simulink model "C3_Stationary_Exp"  (R2019a)
settings: Solver=VariableStepAuto  StartTime=0.0  StopTime=10.0  RelTol=1e-3
values from neighbouring files (symbols this model uses):
  a =     [C2_Preliminary_Controller_Design.m]    (also in D1_Preliminary_Controller_Design.m = 0.199; D2_Controller_Design.m = 0.199; D3_PL_Controller_Design.m = 0.199; D4_DPDZ_Controller_Design.m = 0.199)
  g = 9.81    [C2_Preliminary_Controller_Design.m]    (also in D1_Preliminary_Controller_Design.m; D2_Controller_Design.m; D3_PL_Controller_Design.m; D4_DPDZ_Controller_Design.m)
  h =     [C2_Preliminary_Controller_Design.m]    (also in D1_Preliminary_Controller_Design.m = 0.0966; D2_Controller_Design.m = 0.0966; D3_PL_Controller_Design.m = 0.0966; D4_DPDZ_Controller_Design.m = 0.0966)
  sine_lambda = sin(lambda)    [C2_Preliminary_Controller_Design.m]    (also in D1_Preliminary_Controller_Design.m; D2_Controller_Design.m; D3_PL_Controller_Design.m; D4_DPDZ_Controller_Design.m)
settings Model: Creator=Conor  LastModifiedBy=Conor

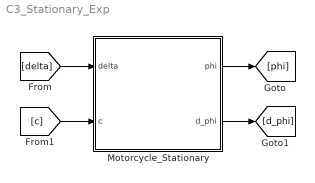
== system C3_Stationary_Exp ==
  Motorcycle_Stationary : Subsystem
  wires:
  Motorcycle_Stationary/1(phi) -> [phi]
  [c] -> Motorcycle_Stationary/2(c)
  [delta] -> Motorcycle_Stationary/1(delta)
  Motorcycle_Stationary/2(d_phi) -> [d_phi]

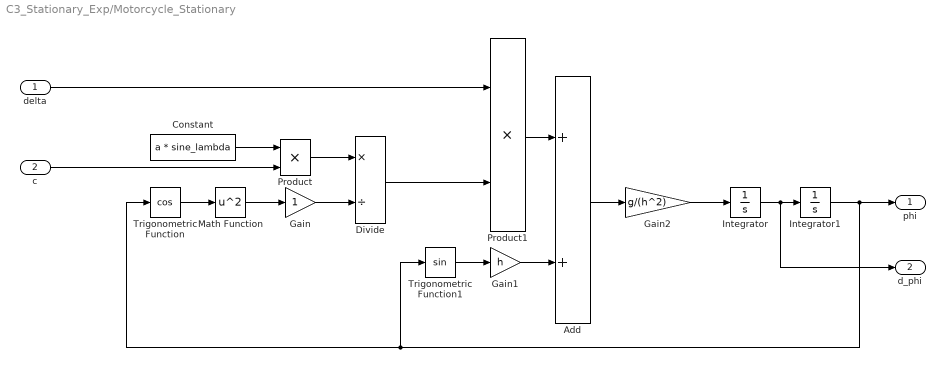
== system C3_Stationary_Exp/Motorcycle_Stationary ==
  delta : Inport
  c : Inport  Port=2
  Add : Sum
  Constant : Constant  Value=a * sine_lambda
  Divide : Product  Inputs=*/
  Gain : Gain
  Gain1 : Gain  Gain=h
  Gain2 : Gain  Gain=g/(h^2)
  Integrator : Integrator
  Integrator1 : Integrator
  Math Function : Math  Operator=square  SaturateOnIntegerOverflow=on
  Product : Product
  Product1 : Product
  Trigonometric Function : Trigonometry  Operator=cos
  Trigonometric Function1 : Trigonometry
  phi : Outport
  d_phi : Outport  Port=2
  wires:
  c/1 -> Product/2
  Constant/1 -> Product/1
  Product/1 -> Divide/1
  Gain/1 -> Divide/2
  Math Function/1 -> Gain/1
  Trigonometric Function/1 -> Math Function/1
  Divide/1 -> Product1/2
  delta/1 -> Product1/1
  Product1/1 -> Add/1
  Gain1/1 -> Add/2
  Trigonometric Function1/1 -> Gain1/1
  Add/1 -> Gain2/1
  Gain2/1 -> Integrator/1
  Integrator/1 -> d_phi/1, Integrator1/1
  Integrator1/1 -> Trigonometric Function1/1, Trigonometric Function/1, phi/1
